simulink model "MPC_THE_ONE_TO_USE"  (R2020a)
settings: Solver=FixedStepAuto  StartTime=0.0  StopTime=15  FixedStep=1e-1  RelTol=1e-3
values from neighbouring files (symbols this model uses):
  l = 0.25    [init.m]    (also in matlab.mat)
libraries: mpclib x1, cstblocks x1

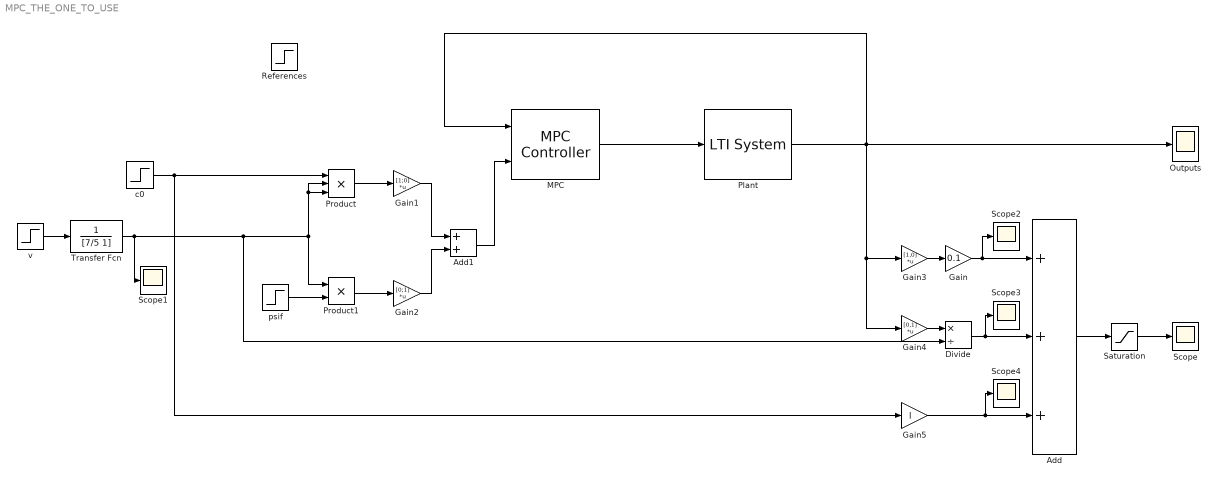
== system MPC_THE_ONE_TO_USE ==
  Add : Sum  Inputs=+++
  Add1 : Sum
  Divide : Product  Inputs=*/
  Gain : Gain  Gain=0.1
  Gain1 : Gain  Gain=[1;0]  Multiplication=Matrix(K*u)
  Gain2 : Gain  Gain=[0;1]  Multiplication=Matrix(K*u)
  Gain3 : Gain  Gain=[1,0]  Multiplication=Matrix(K*u)
  Gain4 : Gain  Gain=[0,1]  Multiplication=Matrix(K*u)
  Gain5 : Gain  Gain=l
  MPC : mpclib/MPC Controller  SCDEnableBlockLinearizationSpecification=on  mpcobj=mpc1_C  is_multiple=0  enable_value=0  return_u0=off  updateMPCinCallerWorkspace=on  md_inport=off  mv_inport=off  uref_inport=off  return_cost=off  return_mvseq=off  return_qpstatus=off  return_xseq=off  return_state=off  return_ovseq=off  state_inport=off  umin_inport=off  umax_inport=off  ymin_inport=off  ymax_inport=off  cc_inport=off  ywt_inport=off  uwt_inport=off  duwt_inport=off  rhoeps_inport=off  pm_inport=off  MaximumP=10  HorizonChoice=FixedHorizon  n_ts=0.1  n_p=10  n_mv=2  n_md=0  n_ud=0  n_mo=2  n_uo=0  BlockDataType=double  SampleTimeInherited=off  switch_inport=off
  Outputs : Scope
  Plant : cstblocks/LTI System  sys=mpc1_G  IC=[]
  Product : Product  Inputs=3
  Product1 : Product
  References : Step  Before=[0;0]  After=[1;1]
  Saturation : Saturate  UpperLimit=inf  LowerLimit=-inf
  Scope{,1..4} (5 alike) : Scope
  Transfer Fcn : TransferFcn  Denominator=[7/5 1]
  c0 : Step  SampleTime=0
  psif : Step  SampleTime=0
  v : Step  Time=0.2  SampleTime=0
  wires:
  MPC/1 -> Plant/1
  c0/1 -> Gain5/1, Product/1
  v/1 -> Transfer Fcn/1
  psif/1 -> Product1/2
  Gain/1 -> Scope2/1, Add/1
  Divide/1 -> Scope3/1, Add/2
  Add/1 -> Saturation/1
  Gain1/1 -> Add1/1
  Gain2/1 -> Add1/2
  Product1/1 -> Gain2/1
  Product/1 -> Gain1/1
  Add1/1 -> MPC/2
  Gain3/1 -> Gain/1
  Gain4/1 -> Divide/1
  Gain5/1 -> Scope4/1, Add/3
  Saturation/1 -> Scope/1
  Transfer Fcn/1 -> Scope1/1, Divide/2, Product1/1, Product/3, Product/2
  Plant/1 -> Outputs/1, MPC/1, Gain4/1, Gain3/1
